simulink model "s6"  (Simulink 2.00)
settings: Solver=ode15s  StartTime=0.0  StopTime=tstop  MaxStep=1e-2  RelTol=1e-6  AbsTol=1e-6
values from neighbouring files (symbols this model uses):
  Caprun = 1    [M6.M]
  Capstart = 0    [M6.M]
  Crun = -1/(wb*Xcrun)    [M6.M]
  Cstart = -1/(wb*Xcstart)    [M6.M]
  Domega = 0    [P1HP.M]    (also in PSPH.M)
  H = J*wbm*wbm/(2*Sb)    (= 2.36870505626)    [P1HP.M]    (also in PSPH.M = 1.39074103839)
  Nq2Nd = 1/1.18    (= 0.847457627119)    [PSPH.M]
  Psipdro = 0    [M1.M]    (also in M4.M; M4STP.M; M5.M; M6.M)
  Psipdso = 0    [M6.M]
  Psipqro = 0    [M1.M]    (also in M4.M = Vm; M4STP.M = Vm; M5.M; M6.M)
  Psiqso = 0    [M1.M]    (also in M4.M = Vm; M4STP.M = Vm; M5.M; M6.M)
  Rcrun = real(zpcrun)    [M6.M]
  Rcstart = real(zpcstart)    [M6.M]
  rpds = (Nq2Nd^2)*rds    (= 5.1278368285)    [PSPH.M]
  rpr = 1.99    [P1HP.M]    (also in PSPH.M = 4.12)
  rqs = 2.02    [PSPH.M]
  Tfactor = (3*P)/(4*wb)    (= 0.00795774715459)    [P1HP.M]    (also in PSPH.M = 0.00530516476973)
  tmech_time = [0 0.8 0.8 1.2 1.2 1.6 1.6 tstop]    [M1.M]    (also in M6.M = [0 1.5 1.5 1.75 1.75 2.0 2.0 2.25 2.25 2.5])
  tmech_value = [0 0 -0.5 -0.5 -1. -1. -0.5 -0.5]*Tb    [M1.M]    (also in M6.M = [0 0 -Tb -Tb -Tb/2 -Tb/2 -Tb -Tb 0 0 ])
  Vm = Vrated*sqrt(2/3)    [M4.M]    (also in P1HP.M; PSPH.M = Vrated*sqrt(2))
  wb = 2*pi*frated    (= 376.991118431)    [P1HP.M]    (also in PSPH.M)
  we = wb    (= 376.991118431)    [P1HP.M]    (also in PSPH.M)
  wrbywbo = 0    [M1.M]    (also in M4.M = 1; M4STP.M = 1; M5.M; M6.M)
  wrswbywb = 0.75    [M6.M]
  xlqs = 2.79    [PSPH.M]
  xMd = 1/(1/xmq + 1/xplds + 1/xplr)    (= 1.08803209665)    [PSPH.M]
  xmq = 66.8    [PSPH.M]
  xMq = 1/(1/xmq + 1/xlqs + 1/xplr)    (= 1.18330436283)    [PSPH.M]
  xplds = (Nq2Nd^2)*xlds    (= 2.31255386383)    [PSPH.M]
  xplr = xls    (= 2.61631836191)    [P1HP.M]    (also in PSPH.M = 2.12)
settings Model: SaveTime=off  SaveOutput=off  ConsistencyChecking=off

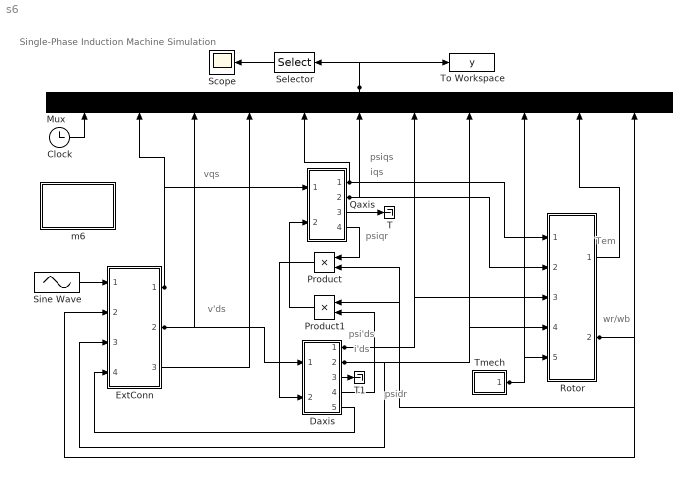
== system s6 ==
  note: Single-Phase Induction
      | Machine Simulation
  note: Tem
  note: wr/wb
  note: psi'ds
  note: i'ds
  note: iqs
  note: psiqs
  note: v'ds
  note: vqs
  note: psiqr
  note: psidr
  Clock : Clock
      settings: DeleteFcn=simclock BlockIsBeingDestroyed  PostSaveFcn=simclock Save
  Daxis : Subsystem
  ExtConn : Subsystem
  m6 : Subsystem
      settings: OpenFcn=m6
      mask Type: Masked block of m6.m
      mask Help: Uses m6.m to initialize and plot
      mask Display: disp('Initialize\nand plot')
  Mux : Mux  Orientation=up  Inputs=11
  Product : Product  Orientation=left  Inputs=2
  Product1 : Product  Orientation=left  Inputs=2
  Qaxis : Subsystem
  Rotor : Subsystem
  Scope : Scope
      settings: TickLabels=on  TimeRange=auto  YMin=-5  YMax=5  SaveToWorkspace=off  SaveName=ScopeData  LimitMaxRows=off
  Selector : Selector  Orientation=left  Elements=[2 3 5 7 10 11]  InputPortWidth=11
  Sine Wave : Sin  Amplitude=Vm  Frequency=we  Phase=-pi/2  SampleTime=-1
  T : Terminator
  T1 : Terminator
  Tmech : Subsystem  mask(Repeating table){rep_seq_t=tmech_time, rep_seq_y=tmech_value}
      mask prompts: rep_seq_t "Time values:"; rep_seq_y "Output values:"
      mask help: Repeating table.
      mask init:
      | period = max(rep_seq_t);
      mask Help: Repeats cycle given in table. Time values should be monotonically increasing.
      mask Display: plot([rep_seq_t,rep_seq_t+period,rep_seq_t+2*period,rep_seq_t(1)+3*period],[rep_seq_y,rep_seq_y,rep_seq_y,rep_seq_y(1)])
  To Workspace : ToWorkspace  VariableName=y  SampleTime=0
      settings: Buffer=80000
  wires:
  Daxis/3(out_idr') -> T1/1
  Qaxis/3(out_iqr') -> T/1
  ExtConn/3(out_Vcap) -> Mux/4
  Rotor/1(out_Tem) -> Mux/10
  Clock/1 -> Mux/1
  Daxis/5(out_dpsidr'/dt) -> ExtConn/4(in_dpsidr'/dt)
  Qaxis/1(out_psiqs) -> Mux/5, Rotor/1(in_psiqs)
  Qaxis/2(out_iqs) -> Mux/6, Rotor/2(in_iqs)
  Daxis/1(out_psi'ds) -> Mux/7, Rotor/3(in_psi'ds)
  Tmech/1(out_1) -> Mux/9, Rotor/5(in_Tmech)
  ExtConn/2(out_v'ds) -> Mux/3, Daxis/1(in_v'ds)
  ExtConn/1(out_vqs) -> Mux/2, Qaxis/1(in_vqs)
  Sine Wave/1 -> ExtConn/1(in_vas)
  Daxis/2(out_i'ds) -> Mux/8, ExtConn/3(in_i'ds), Rotor/4(in_i'ds)
  Daxis/4(out_psidr') -> Product1/2
  Qaxis/4(out_psiqr') -> Product/1
  Rotor/2(out_wr/wb) -> Mux/11, ExtConn/2(in_wr/wb), Product1/1, Product/2
  Product/1 -> Daxis/2(in_(wr/wb)*psiqr')
  Product1/1 -> Qaxis/2(in_(wr/wb)*psidr')
  Mux/1 -> To Workspace/1, Selector/1
  Selector/1 -> Scope/1

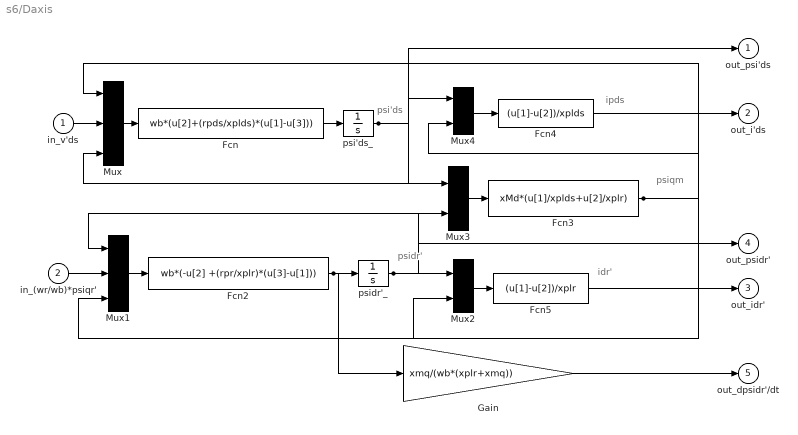
== system s6/Daxis ==
  note: psidr'
  note: psi'ds
  note: ipds
  note: idr'
  note: psiqm
  in_v'ds : Inport  Port=1  PortWidth=-1  SampleTime=-1
  in_(wr/wb)*psiqr' : Inport  Port=2  PortWidth=-1  SampleTime=-1
  Fcn : Fcn  Expr=wb*(u[2]+(rpds/xplds)*(u[1]-u[3]))
  Fcn2 : Fcn  Expr=wb*(-u[2] +(rpr/xplr)*(u[3]-u[1]))
  Fcn3 : Fcn  Expr=xMd*(u[1]/xplds+u[2]/xplr)
  Fcn4 : Fcn  Expr=(u[1]-u[2])/xplds
  Fcn5 : Fcn  Expr=(u[1]-u[2])/xplr
  Gain : Gain  Gain=xmq/(wb*(xplr+xmq))
  Mux : Mux  Inputs=3
  Mux1 : Mux  Inputs=3
  Mux2 : Mux  Inputs=2
  Mux3 : Mux  Inputs=2
  Mux4 : Mux  Inputs=2
  psi'ds_ : Integrator  ExternalReset=none  InitialConditionSource=internal  InitialCondition=Psipdso  LimitOutput=off  UpperSaturationLimit=inf  LowerSaturationLimit=-inf  ShowSaturationPort=off  ShowStatePort=off  AbsoluteTolerance=auto
  psidr'_ : Integrator  ExternalReset=none  InitialConditionSource=internal  InitialCondition=Psipdro  LimitOutput=off  UpperSaturationLimit=inf  LowerSaturationLimit=-inf  ShowSaturationPort=off  ShowStatePort=off  AbsoluteTolerance=auto
  out_psi'ds : Outport  Port=1  InitialOutput=0
  out_i'ds : Outport  Port=2  InitialOutput=0
  out_idr' : Outport  Port=3  InitialOutput=0
  out_psidr' : Outport  Port=4  InitialOutput=0
  out_dpsidr'/dt : Outport  Port=5  InitialOutput=0
  wires:
  Fcn2/1 -> Gain/1, psidr'_/1
  Gain/1 -> out_dpsidr'/dt/1
  Fcn5/1 -> out_idr'/1
  in_(wr/wb)*psiqr'/1 -> Mux1/2
  in_v'ds/1 -> Mux/2
  Fcn4/1 -> out_i'ds/1
  Mux/1 -> Fcn/1
  Fcn/1 -> psi'ds_/1
  Mux3/1 -> Fcn3/1
  Mux4/1 -> Fcn4/1
  psi'ds_/1 -> out_psi'ds/1, Mux3/1, Mux4/1, Mux/3
  Fcn3/1 -> Mux4/2, Mux1/3, Mux/1, Mux2/2
  Mux1/1 -> Fcn2/1
  psidr'_/1 -> out_psidr'/1, Mux1/1, Mux3/2, Mux2/1
  Mux2/1 -> Fcn5/1

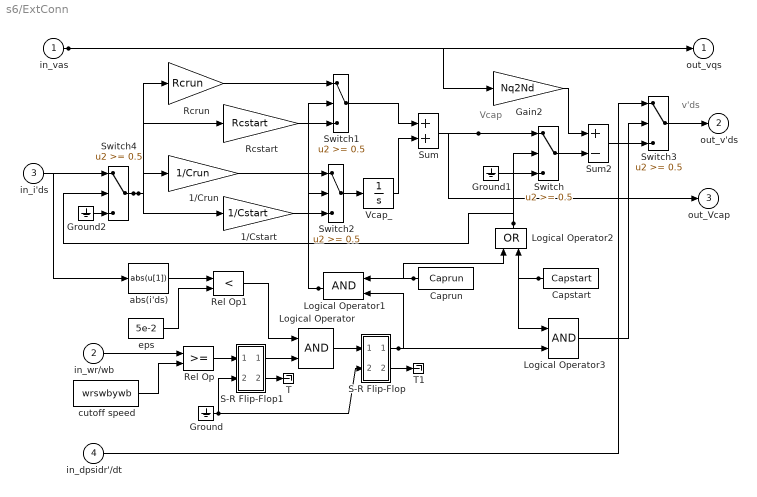
== system s6/ExtConn ==
  note: v'ds
  note: Vcap
  in_vas : Inport  Port=1  PortWidth=-1  SampleTime=-1
  in_wr/wb : Inport  Port=2  PortWidth=-1  SampleTime=-1
  in_i'ds : Inport  Port=3  PortWidth=-1  SampleTime=-1
  in_dpsidr'/dt : Inport  Port=4  PortWidth=-1  SampleTime=-1
  1/Crun : Gain  Gain=1/Crun
  1/Cstart : Gain  Gain=1/Cstart
  Caprun : Constant  Orientation=left  Value=Caprun
  Capstart : Constant  Orientation=left  Value=Capstart
  Gain2 : Gain  Gain=Nq2Nd
  Ground : Ground
  Ground1 : Ground
  Ground2 : Ground
  Logical Operator : Logic  Operator=AND  Inputs=2
  Logical Operator1 : Logic  Orientation=left  Operator=AND  Inputs=2
  Logical Operator2 : Logic  Orientation=up  Operator=OR  Inputs=2
  Logical Operator3 : Logic  Operator=AND  Inputs=2
  Rcrun : Gain  Gain=Rcrun
  Rcstart : Gain  Gain=Rcstart
  Rel Op : RelationalOperator  Operator=>=
  Rel Op1 : RelationalOperator  Operator=<
  S-R Flip-Flop : Subsystem
  S-R Flip-Flop1 : Subsystem
  Sum : Sum  Inputs=++
  Sum2 : Sum  Inputs=+-
  Switch{,1..4} (5 alike) : Switch  Threshold=0.5
  T : Terminator
  T1 : Terminator
  Vcap_ : Integrator  ExternalReset=none  InitialConditionSource=internal  InitialCondition=0  LimitOutput=off  UpperSaturationLimit=inf  LowerSaturationLimit=-inf  ShowSaturationPort=off  ShowStatePort=off  AbsoluteTolerance=auto
  abs(i'ds) : Fcn  Expr=abs(u[1])
  cutoff speed : Constant  Value=wrswbywb
  eps : Constant  Value=5e-2
  out_vqs : Outport  Port=1  InitialOutput=0
  out_v'ds : Outport  Port=2  InitialOutput=0
  out_Vcap : Outport  Port=3  InitialOutput=0
  wires:
  Sum/1 -> Switch/1, out_Vcap/1
  Switch/1 -> Sum2/2
  Logical Operator2/1 -> Switch4/2, Switch/2
  in_i'ds/1 -> Switch4/1, abs(i'ds)/1
  S-R Flip-Flop/1(Q) -> Logical Operator3/2, Logical Operator1/2
  Capstart/1 -> Logical Operator3/1, Logical Operator2/2
  Caprun/1 -> Logical Operator2/1, Logical Operator1/1
  1/Crun/1 -> Switch2/1
  1/Cstart/1 -> Switch2/3
  Rcrun/1 -> Switch1/1
  Rcstart/1 -> Switch1/3
  Logical Operator1/1 -> Switch1/2, Switch2/2
  Switch1/1 -> Sum/1
  Logical Operator/1 -> S-R Flip-Flop/1(S)
  Rel Op1/1 -> Logical Operator/1
  eps/1 -> Rel Op1/2
  abs(i'ds)/1 -> Rel Op1/1
  cutoff speed/1 -> Rel Op/2
  in_wr/wb/1 -> Rel Op/1
  Gain2/1 -> Sum2/1
  in_vas/1 -> Gain2/1, out_vqs/1
  Ground1/1 -> Switch/3
  Ground2/1 -> Switch4/3
  in_dpsidr'/dt/1 -> Switch3/1
  Sum2/1 -> Switch3/3
  Logical Operator3/1 -> Switch3/2
  Switch3/1 -> out_v'ds/1
  Vcap_/1 -> Sum/2
  Switch2/1 -> Vcap_/1
  Switch4/1 -> Rcrun/1, 1/Cstart/1, Rcstart/1, 1/Crun/1
  S-R Flip-Flop/2(!Q) -> T1/1
  S-R Flip-Flop1/1(Q) -> Logical Operator/2
  Rel Op/1 -> S-R Flip-Flop1/1(S)
  Ground/1 -> S-R Flip-Flop/2(R), S-R Flip-Flop1/2(R)
  S-R Flip-Flop1/2(!Q) -> T/1

== system s6/m6 ==
  note: Masked block of m6.m to initialize s6.m
      | and plot results

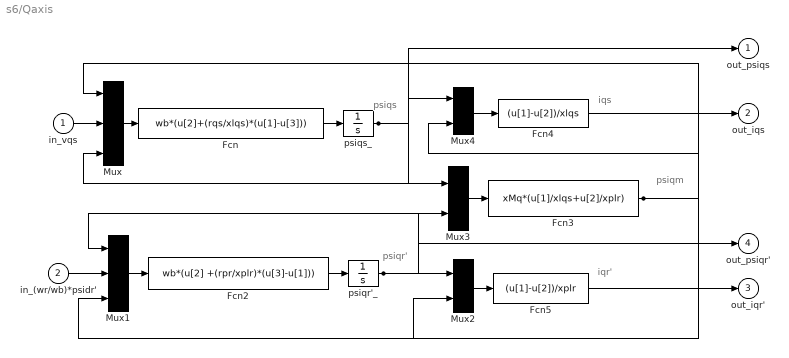
== system s6/Qaxis ==
  note: psiqr'
  note: iqr'
  note: psiqm
  note: psiqs
  note: iqs
  in_vqs : Inport  Port=1  PortWidth=-1  SampleTime=-1
  in_(wr/wb)*psidr' : Inport  Port=2  PortWidth=-1  SampleTime=-1
  Fcn : Fcn  Expr=wb*(u[2]+(rqs/xlqs)*(u[1]-u[3]))
  Fcn2 : Fcn  Expr=wb*(u[2] +(rpr/xplr)*(u[3]-u[1]))
  Fcn3 : Fcn  Expr=xMq*(u[1]/xlqs+u[2]/xplr)
  Fcn4 : Fcn  Expr=(u[1]-u[2])/xlqs
  Fcn5 : Fcn  Expr=(u[1]-u[2])/xplr
  Mux : Mux  Inputs=3
  Mux1 : Mux  Inputs=3
  Mux2 : Mux  Inputs=2
  Mux3 : Mux  Inputs=2
  Mux4 : Mux  Inputs=2
  psiqr'_ : Integrator  ExternalReset=none  InitialConditionSource=internal  InitialCondition=Psipqro  LimitOutput=off  UpperSaturationLimit=inf  LowerSaturationLimit=-inf  ShowSaturationPort=off  ShowStatePort=off  AbsoluteTolerance=auto
  psiqs_ : Integrator  ExternalReset=none  InitialConditionSource=internal  InitialCondition=Psiqso  LimitOutput=off  UpperSaturationLimit=inf  LowerSaturationLimit=-inf  ShowSaturationPort=off  ShowStatePort=off  AbsoluteTolerance=auto
  out_psiqs : Outport  Port=1  InitialOutput=0
  out_iqs : Outport  Port=2  InitialOutput=0
  out_iqr' : Outport  Port=3  InitialOutput=0
  out_psiqr' : Outport  Port=4  InitialOutput=0
  wires:
  Fcn5/1 -> out_iqr'/1
  in_(wr/wb)*psidr'/1 -> Mux1/2
  in_vqs/1 -> Mux/2
  Fcn4/1 -> out_iqs/1
  Mux/1 -> Fcn/1
  Fcn/1 -> psiqs_/1
  Fcn2/1 -> psiqr'_/1
  Mux3/1 -> Fcn3/1
  Mux4/1 -> Fcn4/1
  psiqs_/1 -> out_psiqs/1, Mux3/1, Mux4/1, Mux/3
  Fcn3/1 -> Mux4/2, Mux1/3, Mux/1, Mux2/2
  Mux1/1 -> Fcn2/1
  psiqr'_/1 -> out_psiqr'/1, Mux1/1, Mux3/2, Mux2/1
  Mux2/1 -> Fcn5/1

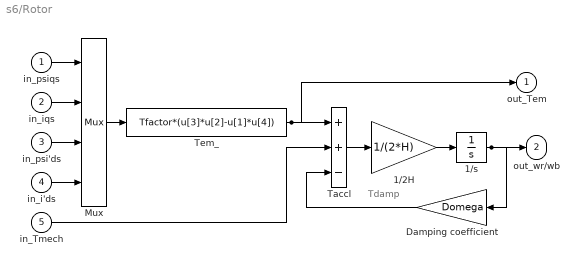
== system s6/Rotor ==
  note: Tdamp
  in_psiqs : Inport  Port=1  PortWidth=-1  SampleTime=-1
  in_iqs : Inport  Port=2  PortWidth=-1  SampleTime=-1
  in_psi'ds : Inport  Port=3  PortWidth=-1  SampleTime=-1
  in_i'ds : Inport  Port=4  PortWidth=-1  SampleTime=-1
  in_Tmech : Inport  Port=5  PortWidth=-1  SampleTime=-1
  1/2H : Gain  Gain=1/(2*H)
  1/s : Integrator  ExternalReset=none  InitialConditionSource=internal  InitialCondition=wrbywbo  LimitOutput=off  UpperSaturationLimit=inf  LowerSaturationLimit=-inf  ShowSaturationPort=off  ShowStatePort=off  AbsoluteTolerance=auto
  Damping coefficient : Gain  Orientation=left  Gain=Domega
  Mux : Mux  Inputs=4
  Taccl : Sum  Inputs=++-
  Tem_ : Fcn  Expr=Tfactor*(u[3]*u[2]-u[1]*u[4])
  out_Tem : Outport  Port=1  InitialOutput=0
  out_wr/wb : Outport  Port=2  InitialOutput=0
  wires:
  in_i'ds/1 -> Mux/4
  in_psi'ds/1 -> Mux/3
  in_iqs/1 -> Mux/2
  in_psiqs/1 -> Mux/1
  Mux/1 -> Tem_/1
  Damping coefficient/1 -> Taccl/3
  1/s/1 -> Damping coefficient/1, out_wr/wb/1
  Tem_/1 -> out_Tem/1, Taccl/1
  1/2H/1 -> 1/s/1
  Taccl/1 -> 1/2H/1
  in_Tmech/1 -> Taccl/2

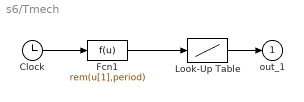
== system s6/Tmech ==
  Clock : Clock
      settings: DeleteFcn=simclock BlockIsBeingDestroyed  PostSaveFcn=simclock Save
  Fcn1 : Fcn  Expr=rem(u[1],period)
  Look-Up Table : Lookup  InputValues=rep_seq_t  OutputValues=rep_seq_y
  out_1 : Outport  Port=1  InitialOutput=0
  wires:
  Look-Up Table/1 -> out_1/1
  Clock/1 -> Fcn1/1
  Fcn1/1 -> Look-Up Table/1

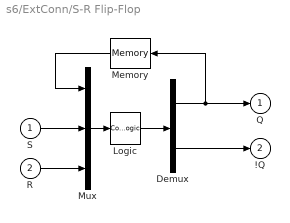
== system s6/ExtConn/S-R Flip-Flop ==
  S : Inport  Port=1  PortWidth=-1  SampleTime=-1
  R : Inport  Port=2  PortWidth=-1  SampleTime=-1
  Demux : Demux  Outputs=2
  Logic : CombinatorialLogic  TruthTable=[0 1;0 1;1 0;0 1;1 0;0 1;1 0;1 0]
  Memory : Memory  Orientation=left  X0=0  InheritSampleTime=on
  Mux : Mux  Inputs=3
  Q : Outport  Port=1  InitialOutput=0
  !Q : Outport  Port=2  InitialOutput=1
  wires:
  R/1 -> Mux/3
  S/1 -> Mux/2
  Memory/1 -> Mux/1
  Demux/1 -> Memory/1, Q/1
  Demux/2 -> !Q/1
  Logic/1 -> Demux/1
  Mux/1 -> Logic/1

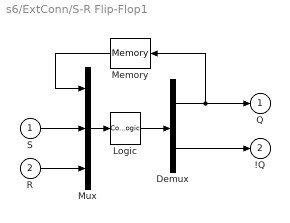
== system s6/ExtConn/S-R Flip-Flop1 ==
  S : Inport  Port=1  PortWidth=-1  SampleTime=-1
  R : Inport  Port=2  PortWidth=-1  SampleTime=-1
  Demux : Demux  Outputs=2
  Logic : CombinatorialLogic  TruthTable=[0 1;0 1;1 0;0 1;1 0;0 1;1 0;1 0]
  Memory : Memory  Orientation=left  X0=0  InheritSampleTime=on
  Mux : Mux  Inputs=3
  Q : Outport  Port=1  InitialOutput=0
  !Q : Outport  Port=2  InitialOutput=1
  wires:
  R/1 -> Mux/3
  S/1 -> Mux/2
  Memory/1 -> Mux/1
  Demux/1 -> Memory/1, Q/1
  Demux/2 -> !Q/1
  Logic/1 -> Demux/1
  Mux/1 -> Logic/1
